simulink model "clasificador"  (Simulink 7.5)
settings: Solver=ode45  StartTime=0.0  StopTime=10.0  RelTol=1e-3
libraries: neural x12
settings Model: Creator=José  LastModifiedBy=José

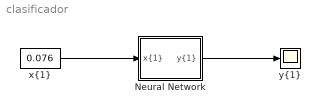
== system clasificador ==
  Neural Network : Subsystem
  "x{1}" : Constant  Value=0.076
      mask Display: disp('Input 1 ')
  "y{1}" : Scope
      settings: DataFormat=Array
  wires:
  "x{1}"/1 -> Neural Network/1("x{1}")
  Neural Network/1("y{1}") -> "y{1}"/1

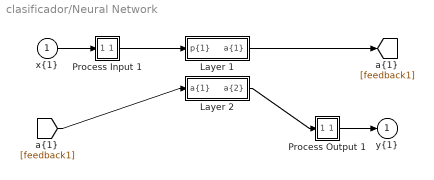
== system clasificador/Neural Network ==
  "x{1}" : Inport  PortDimensions=1  SampleTime=1
  Layer 1 : Subsystem
  Layer 2 : Subsystem
  Process Input 1 : Subsystem
  Process Output 1 : Subsystem
  "y{1}" : Outport  InitialOutput=[0;0;0]
  wires:
  "x{1}"/1 -> Process Input 1/1(x)
  Process Output 1/1(y) -> "y{1}"/1
  Process Input 1/1(p) -> Layer 1/1("p{1}")
  Layer 1/1("a{1}") -> [feedback1]
  [feedback1] -> Layer 2/1("a{1} ")
  Layer 2/1("a{2}") -> Process Output 1/1(a)

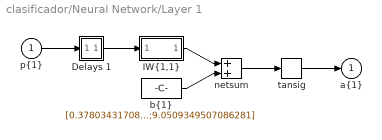
== system clasificador/Neural Network/Layer 1 ==
  "p{1}" : Inport  PortDimensions=1  SampleTime=1
  Delays 1 : Subsystem
      mask Display: disp('TDL')
  "IW{1,1}" : Subsystem
      mask Display: disp('weight')
  "b{1}" : Constant  Value=[0.3780343170820849;9.0509349507086281]
      mask Display: disp('bias')
  netsum : Sum  Inputs=2  OutDataType=sfix(16)  OutScaling=2^0  SaturateOnIntegerOverflow=on  InputSameDT=on  OutDataTypeStr=Inherit: Same as first input
  tansig : neural/Transfer Functions/tansig  SystemSampleTime=-1
  "a{1}" : Outport  InitialOutput=[0;0]
  wires:
  "p{1}"/1 -> Delays 1/1("p{1}")
  Delays 1/1("pd{1,1}") -> "IW{1,1}"/1("pd{1,1}")
  "IW{1,1}"/1("iz{1,1}") -> netsum/1
  "b{1}"/1 -> netsum/2
  netsum/1 -> tansig/1
  tansig/1 -> "a{1}"/1

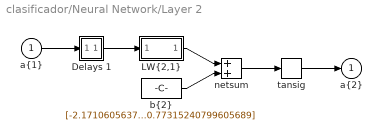
== system clasificador/Neural Network/Layer 2 ==
  "a{1} " : Inport  PortDimensions=2  SampleTime=1
  Delays 1 : Subsystem
      mask Display: disp('TDL')
  "LW{2,1}" : Subsystem
      mask Display: disp('weight')
  "b{2}" : Constant  Value=[-2.1710605637544158;-12.718007534691328;-0.77315240799605689]
      mask Display: disp('bias')
  netsum : Sum  Inputs=2  OutDataType=sfix(16)  OutScaling=2^0  SaturateOnIntegerOverflow=on  InputSameDT=on  OutDataTypeStr=Inherit: Same as first input
  tansig : neural/Transfer Functions/tansig  SystemSampleTime=-1
  "a{2}" : Outport  InitialOutput=[0;0;0]
  wires:
  "a{1} "/1 -> Delays 1/1("p{2}")
  Delays 1/1("pd{2,1}") -> "LW{2,1}"/1("ad{2,1}")
  "LW{2,1}"/1("lz{2,1}") -> netsum/1
  "b{2}"/1 -> netsum/2
  netsum/1 -> tansig/1
  tansig/1 -> "a{2}"/1

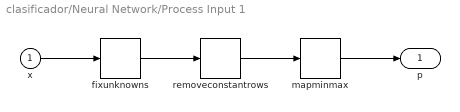
== system clasificador/Neural Network/Process Input 1 ==
  x : Inport  PortDimensions=1  SampleTime=1
  fixunknowns : neural/Processing Functions/fixunknowns  SystemSampleTime=-1  dummy=0
  mapminmax : neural/Processing Functions/mapminmax  SystemSampleTime=-1  xmin=13.764959  xmax=24.695869  ymin=-1  ymax=1
  removeconstantrows : neural/Processing Functions/removeconstantrows  SystemSampleTime=-1  inputSize=1  keep=1
  p : Outport  PortDimensions=1  SampleTime=1
  wires:
  x/1 -> fixunknowns/1
  fixunknowns/1 -> removeconstantrows/1
  removeconstantrows/1 -> mapminmax/1
  mapminmax/1 -> p/1

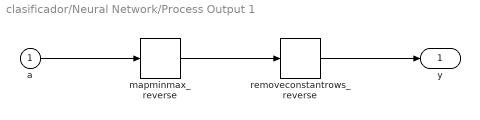
== system clasificador/Neural Network/Process Output 1 ==
  a : Inport  PortDimensions=3  SampleTime=1
  mapminmax_reverse : neural/Processing Functions/mapminmax_reverse  SystemSampleTime=-1  xmin=[0;0;0]  xmax=[1;1;1]  ymin=-1  ymax=1
  removeconstantrows_reverse : neural/Processing Functions/removeconstantrows_reverse  SystemSampleTime=-1  inputSize=3  constants=zeros(0,1)  rearrange=[1 2 3]
  y : Outport  PortDimensions=3  SampleTime=1
  wires:
  a/1 -> mapminmax_reverse/1
  mapminmax_reverse/1 -> removeconstantrows_reverse/1
  removeconstantrows_reverse/1 -> y/1

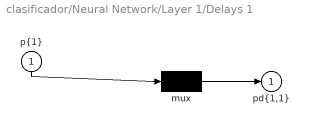
== system clasificador/Neural Network/Layer 1/Delays 1 ==
  "p{1}" : Inport  PortDimensions=1  SampleTime=1
  mux : Mux  Inputs=1
  "pd{1,1}" : Outport
  wires:
  "p{1}"/1 -> mux/1
  mux/1 -> "pd{1,1}"/1

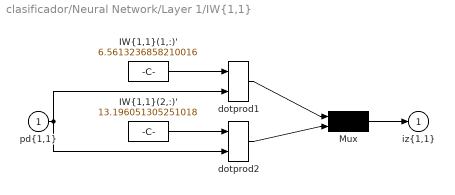
== system clasificador/Neural Network/Layer 1/IW{1,1} ==
  "pd{1,1}" : Inport  PortDimensions=1  SampleTime=1
  "IW{1,1}(1,:)'" : Constant  Value=6.5613236858210016
      mask Display: disp('weights')
  "IW{1,1}(2,:)'" : Constant  Value=13.196051305251018
      mask Display: disp('weights')
  Mux : Mux  Inputs=2
  dotprod1 : neural/Weight Functions/dotprod  SystemSampleTime=-1
  dotprod2 : neural/Weight Functions/dotprod  SystemSampleTime=-1
  "iz{1,1}" : Outport
  wires:
  "IW{1,1}(1,:)'"/1 -> dotprod1/1
  "pd{1,1}"/1 -> dotprod1/2, dotprod2/2
  dotprod1/1 -> Mux/1
  "IW{1,1}(2,:)'"/1 -> dotprod2/1
  dotprod2/1 -> Mux/2
  Mux/1 -> "iz{1,1}"/1

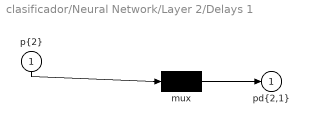
== system clasificador/Neural Network/Layer 2/Delays 1 ==
  "p{2}" : Inport  PortDimensions=2  SampleTime=1
  mux : Mux  Inputs=1
  "pd{2,1}" : Outport
  wires:
  "p{2}"/1 -> mux/1
  mux/1 -> "pd{2,1}"/1

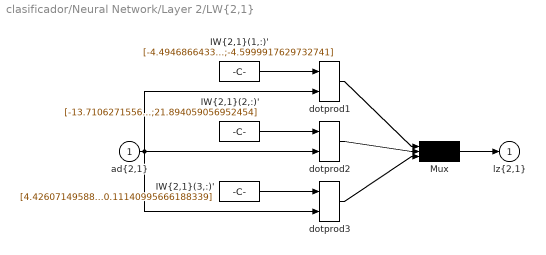
== system clasificador/Neural Network/Layer 2/LW{2,1} ==
  "ad{2,1}" : Inport  PortDimensions=2  SampleTime=1
  "IW{2,1}(1,:)'" : Constant  Value=[-4.4946866433647212;-4.5999917629732741]
      mask Display: disp('weights')
  "IW{2,1}(2,:)'" : Constant  Value=[-13.710627155623156;21.894059056952454]
      mask Display: disp('weights')
  "IW{2,1}(3,:)'" : Constant  Value=[4.4260714958829226;-0.11140995666188339]
      mask Display: disp('weights')
  Mux : Mux  Inputs=3
  dotprod1 : neural/Weight Functions/dotprod  SystemSampleTime=-1
  dotprod2 : neural/Weight Functions/dotprod  SystemSampleTime=-1
  dotprod3 : neural/Weight Functions/dotprod  SystemSampleTime=-1
  "lz{2,1}" : Outport
  wires:
  "IW{2,1}(1,:)'"/1 -> dotprod1/1
  "ad{2,1}"/1 -> dotprod1/2, dotprod2/2, dotprod3/2
  dotprod1/1 -> Mux/1
  "IW{2,1}(2,:)'"/1 -> dotprod2/1
  dotprod2/1 -> Mux/2
  "IW{2,1}(3,:)'"/1 -> dotprod3/1
  dotprod3/1 -> Mux/3
  Mux/1 -> "lz{2,1}"/1
